simulink model "Robot_simulation2"  (R2025b)
settings: Solver=ode15s  StartTime=0.0  StopTime=Tf  FixedStep=dt  RelTol=1e-3
InitFcn:
  | run("init.m");
values from neighbouring files (symbols this model uses):
  dt = 0.1    [init.m]
  F_max = 1500    [init.m]
  F_min = 100    [init.m]
  g = in3(:,13)    [dinamica_3R_numerica.m]    (also in init.m = 9.81)
  k_d = diag([1000, 1000])    [init.m]
  k_p = diag([20000, 20000])    [init.m]
  L_max = 1.2    [init.m]
  mb = 66.5    [init.m]
  mu = 0.6    [init.m]
  N = 5    [init.m]
  q_init = cinematica_inversa_2R(0 , 0.6, robot_params)    [init.m]
  S_bar = 10*kron(eye(N), S)    [init.m]
  W_bar = kron(eye(N), W)    [init.m]
  x_ref = zeros(4, steps)    [init.m]
  x_ref_global = x_ref    [init.m]
undefined symbols (not defined in the file or in its folder): robot_params
libraries: simulink x2, slpidlib x1
settings Model: Creator=Acer  LastModifiedBy=Acer

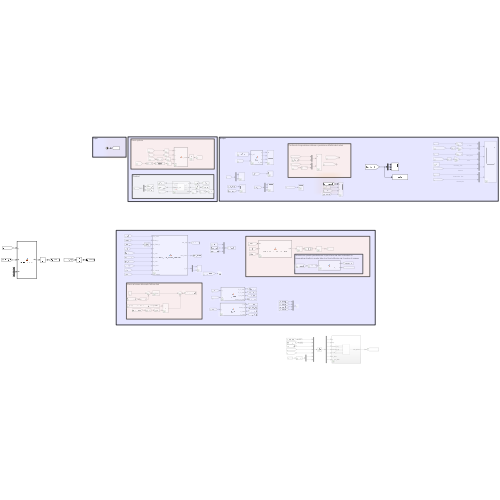
[thumbnail: Simulink's stored preview of the top-level diagram]
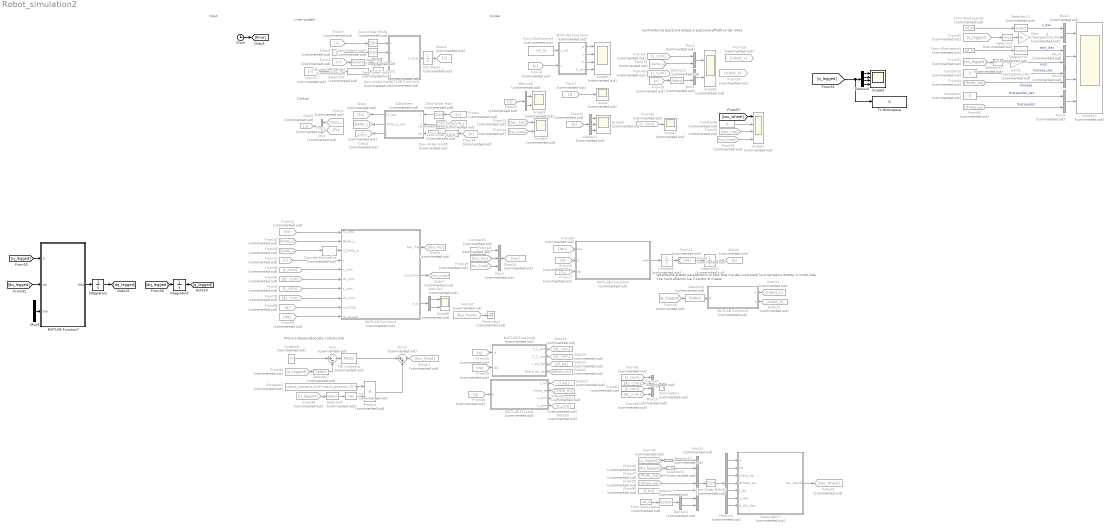
== system Robot_simulation2 ==
  note: Provo a tenere bloccato l'ultimo link
  note: Attenzione questo parallelismo lo puoi fare ma devi calcolarti la
      | cinematica diretta in modo tale che l'end effector sia il centro di massa
  note: Confronto tra posizione attesa e posizione effettiva del robot
  note: Control
  note: Liner system
  note: Input
  note: Scope
  Clock : Clock
  Constant{,3..6} (5 alike) : Constant  Commented=on  Value=0
  Constant2 : Constant  Commented=on  Value=robot_params.m3*robot_params.l3 *g
  Demux1 : Demux  Commented=on  Outputs=3
  Demux2 : Demux  Commented=on  Outputs=2
  Demux3 : Demux
  Demux4 : Demux  Commented=on  Outputs=2
  Demux5 : Demux  Commented=on  Outputs=2
  Demux6 : Demux  Commented=on  Outputs=7
  Discrete Derivative : simulink/Discrete/Discrete Derivative  Commented=on  gainval=1.0  ICPrevScaledInput=0.0  OutMin=[]  OutMax=[]  OutDataType=fixdt(1, 16)  OutScaling=2^-10  DoSatur=off
  Discrete Derivative1 : simulink/Discrete/Discrete Derivative  Commented=on  gainval=1.0  ICPrevScaledInput=0.0  OutMin=[]  OutMax=[]  OutDataType=fixdt(1, 16)  OutScaling=2^-10  DoSatur=off
  From : From  Commented=on  GotoTag=Fz
  From Workspace{1..3,5} (4 alike) : FromWorkspace  Commented=on  VariableName=ref_ts
  From{1,10,25,29} (4 alike) : From  Commented=on  GotoTag=Delta_s
  From11 : From  Commented=on  GotoTag=Fz
  From{2..4,6,12,26..28} (8 alike) : From  Commented=on  GotoTag=x
  From13 : From  Commented=on  GotoTag=tau_hip
  From14 : From  Commented=on  GotoTag=tau_knee
  From{15,17,39,69} (4 alike) : From  Commented=on  GotoTag=dq
  From{16,21..22,48,68} (5 alike) : From  Commented=on  GotoTag=q
  From18 : From  Commented=on  GotoTag=tau_hip
  From19 : From  Commented=on  GotoTag=tau_knee
  From20 : From  Commented=on  GotoTag=tau
  From23 : From  Commented=on  GotoTag=robot_x
  From24 : From  Commented=on  GotoTag=robot_h
  From{35..36,38,45,50} (5 alike) : From  Commented=on  GotoTag=q_legged
  From37 : From  Commented=on  GotoTag=tau_head
  From42 : From  Commented=on  GotoTag=s_com
  From{43,53,58,65} (4 alike) : From  Commented=on  GotoTag=z_com
  From46 : From  Commented=on  GotoTag=dq_legged
  From47 : From  Commented=on  GotoTag=theta_eq
  From49 : From  Commented=on  GotoTag=l_eq
  From5 : From  Commented=on  GotoTag=time
  From51 : From  Commented=on  GotoTag=dq_legged
  From54 : From  Commented=on  GotoTag=tau_hip
  From55 : From  Commented=on  GotoTag=tau_knee
  From56 : From  Commented=on  GotoTag=dtheta_eq
  From59 : From  Commented=on  GotoTag=ds_com
  From60 : From  Commented=on  GotoTag=dz_com
  From61 : From  Commented=on  GotoTag=s_com
  From62 : From  Commented=on  GotoTag=ds_com
  From63 : From  Commented=on  GotoTag=dtheta_eq
  From64 : From  Commented=on  GotoTag=theta_eq
  From66 : From  Commented=on  GotoTag=dz_com
  From67 : From  Commented=on  GotoTag=u
  From7 : From  Commented=on  GotoTag=J
  From8 : From  Commented=on  GotoTag=u
  From9 : From  Commented=on  GotoTag=s_com
  Gain : Gain  Commented=on  Gain=robot_params.Rw
  Gain1 : Gain  Commented=on  Gain=robot_params.Rw
  Goto : Goto  Commented=on  GotoTag=Fz
  Goto1 : Goto  Commented=on  GotoTag=Delta_s
  Goto10 : Goto  Commented=on  GotoTag=tau
  Goto11 : Goto  Commented=on  GotoTag=robot_x
  Goto12 : Goto  Commented=on  GotoTag=robot_h
  Goto13 : Goto  Commented=on  GotoTag=tau_head
  Goto16 : Goto  Commented=on  GotoTag=ds_com
  Goto17 : Goto  Commented=on  GotoTag=l_eq
  Goto18 : Goto  Commented=on  GotoTag=theta_eq
  Goto19 : Goto  Commented=on  GotoTag=s_com
  Goto2 : Goto  Commented=on  GotoTag=J
  Goto20 : Goto  Commented=on  GotoTag=z_com
  Goto21 : Goto  Commented=on  GotoTag=dl_eq
  Goto22 : Goto  Commented=on  GotoTag=tau_wheel
  Goto23 : Goto  Commented=on  GotoTag=dtheta_eq
  Goto24 : Goto  Commented=on  GotoTag=dz_com
  Goto4 : Goto  Commented=on  GotoTag=x
  Goto5 : Goto  Commented=on  GotoTag=u
  Goto6 : Goto  Commented=on  GotoTag=tau_hip
  Goto7 : Goto  Commented=on  GotoTag=tau_knee
  Goto8 : Goto  Commented=on  GotoTag=dq
  Goto9 : Goto  Commented=on  GotoTag=q
  Integrator : Integrator  Commented=on  InitialCondition=zeros(3,1)
  Integrator1 : Integrator  Commented=on  InitialCondition=[q_init;0]
  Integrator2 : Integrator  InitialCondition=zeros(4,1)
  Integrator3 : Integrator  InitialCondition=[0;q_init;0]
  MATLAB Function : MATLAB Function  Commented=on  TreatAsAtomicUnit=on
  MATLAB Function1 : MATLAB Function  Commented=on  TreatAsAtomicUnit=on
  MATLAB Function2 : MATLAB Function  Commented=on  TreatAsAtomicUnit=on
  MATLAB Function3 : MATLAB Function  Commented=on  TreatAsAtomicUnit=on
  MATLAB Function4 : MATLAB Function  Commented=on  TreatAsAtomicUnit=on
  MATLAB Function5 : MATLAB Function  Commented=on  TreatAsAtomicUnit=on
  MATLAB Function7 : MATLAB Function  TreatAsAtomicUnit=on
  MATLAB Function8 : MATLAB Function  Commented=on  TreatAsAtomicUnit=on
  Mux{,2..5,8..9} (7 alike) : Mux  Commented=on  Inputs=2
  Mux1 : Mux  Commented=on  Inputs=3
  Mux10 : Mux  Commented=on
  Mux11 : Mux  Commented=on  Inputs=[1 1 1 1 1 1 1]
  Mux6 : Mux  Inputs=[1 1 2]
  PID Controller : slpidlib/PID Controller  Commented=on  Controller=PID  Form=Parallel  TimeDomain=Continuous-time  UseExternalTs=off  SampleTime=-1  IntegratorMethod=Forward Euler  FilterMethod=Forward Euler  ControllerParametersSource=internal  P=10000  I=10  UseKiTs=off  D=10  UseExternalDerivativeSource=off  N=100  UseFilter=on  TunerSelectOption=Frequency Response Based  InitialConditionSource=internal  InitialConditionForIntegrator=0  InitialConditionForFilter=0  DifferentiatorICPrevScaledInput=0  ExternalReset=none  TrackingMode=off  Kt=1  LimitOutput=off  SatLimitsSource=internal  UpperSaturationLimit=inf  LowerSaturationLimit=-inf  LinearizeAsGain=on  AntiWindupMode=none  Kb=1  LimitIntegrator=off  UpperIntegratorSaturationLimit=inf  LowerIntegratorSaturationLimit=-inf  POutMin=[]  POutMax=[]  IOutMin=[]  IOutMax=[]  DOutMin=[]  DOutMax=[]  NOutMin=[]  NOutMax=[]  SumOutMin=[]  SumOutMax=[]  SaturationOutMin=[]  SaturationOutMax=[]  PParamMin=[]  PParamMax=[]  IParamMin=[]  IParamMax=[]  DParamMin=[]  DParamMax=[]  NParamMin=[]  NParamMax=[]  KbParamMin=[]  KbParamMax=[]  KtParamMin=[]  KtParamMax=[]  KbOutMin=[]  KbOutMax=[]  KtOutMin=[]  KtOutMax=[]  IntegratorOutMin=[]  IntegratorOutMax=[]  FilterOutMin=[]  FilterOutMax=[]  SumI1OutMin=[]  SumI1OutMax=[]  SumI2OutMin=[]  SumI2OutMax=[]  SumI3OutMin=[]  SumI3OutMax=[]  SumI4OutMin=[]  SumI4OutMax=[]  SumDOutMin=[]  SumDOutMax=[]  DifferentiatorOutMin=[]  DifferentiatorOutMax=[]  FilterDiffOutCoefMin=[]  FilterDiffOutCoefMax=[]  ReciprocalOutMin=[]  ReciprocalOutMax=[]  SumDenOutMin=[]  SumDenOutMax=[]  SumNumOutMin=[]  SumNumOutMax=[]  DivideOutMin=[]  DivideOutMax=[]  UdiffTsProdOutMin=[]  UdiffTsProdOutMax=[]  NTsProdOutMin=[]  NTsProdOutMax=[]  UintegralTsProdOutMin=[]  UintegralTsProdOutMax=[]  UngainTsProdOutMin=[]  UngainTsProdOutMax=[]  ClampingZeroOutDataTypeStr=Inherit: Inherit via back propagation  ClampingZeroOutMin=[]  ClampingZeroOutMax=[]  FilterDenConstantOutDataTypeStr=Inherit: Inherit via back propagation  FilterDenConstantOutMin=[]  FilterDenConstantOutMax=[]  PCopyOutDataTypeStr=Inherit: Inherit via back propagation  PCopyOutMin=[]  PCopyOutMax=[]  NCopyOutDataTypeStr=Inherit: Inherit via back propagation  NCopyOutMin=[]  NCopyOutMax=[]  IntegratorContinuousStateAttributes=''  IntegratorStateMustResolveToSignalObject=off  IntegratorRTWStateStorageClass=Auto  FilterContinuousStateAttributes=''  FilterStateMustResolveToSignalObject=off  FilterRTWStateStorageClass=Auto  ParallelPVariant=InternalParameters  IdealPVariant=Disabled  IVariant=InternalParameters  DVariant=InternalParameters  IntegratorVariant=Continuous  SatVariant=Disabled  AWVariant=Passthrough  PCopyVariant=Disabled  TRVariant=Disabled  FdbkBlocksVariant=Forward  IdealPFdbkVariant=Disabled  SatFdbkVariant=Disabled  DerivativeFilterVariant=ContFilter  NVariant=InternalParameters  NCopyVariant=Disabled  FilterICVariant=InternalICsFilter  IntegratorICVariant=InternalICs  ExternalResetVariant=Disabled  TRSumVariant=Passthrough  SumFdbkVariant=Disabled  SumVariant=Sum_PID  TsampFilterVariant=InternalTs  TsampNgainVariant=Passthrough  TsampIntegralVariant=Disabled_SignalSpec  ExternalSaturationOutDataTypeStr=Inherit: Same as second input  DerivativeSourceVariant=ErrorSignal  PreIntVariant=InternalPreInt
  Product : Product  Commented=on
  Scope : Scope  Commented=on
      settings: ActiveDisplayYMinimum=-1  ActiveDisplayYMaximum=1
  Scope1 : Scope  Commented=on  NumInputPorts=4
      settings: ActiveDisplayYMinimum=-1  ActiveDisplayYMaximum=1
  Scope10 : Scope  Commented=on  NumInputPorts=4
      settings: ActiveDisplayYMinimum=-17.232872762989807  ActiveDisplayYMaximum=4.2885654585543138  DataLoggingVariableName=ScopeData10
  Scope2 : Scope  Commented=on  NumInputPorts=4
      settings: ActiveDisplayYMinimum=-0.12515032259253614  ActiveDisplayYMaximum=1.1263529033328255  DataLoggingVariableName=ScopeData2
  Scope3 : Scope  NumInputPorts=4
      settings: ActiveDisplayYMinimum=-33.446881867150935  ActiveDisplayYMaximum=300.84907271752644  DataLoggingVariableName=ScopeData3
  Scope{4,6,8..9} (4 alike) : Scope  Commented=on  NumInputPorts=2
      Scope4 settings: ActiveDisplayYMinimum=-277.12659813654608  ActiveDisplayYMaximum=-227.4623965158911  DataLoggingVariableName=ScopeData4
      Scope6 settings: ActiveDisplayYMinimum=-1  ActiveDisplayYMaximum=1  DataLoggingVariableName=ScopeData6
      Scope8 settings: ActiveDisplayYMinimum=-0.17028433513177135  ActiveDisplayYMaximum=0.13336662971669377  DataLoggingVariableName=ScopeData8
      Scope9 settings: ActiveDisplayYMinimum=-0.0048922557383608324  ActiveDisplayYMaximum=0.0030434800856270639  DataLoggingVariableName=ScopeData9
  Scope5 : Scope  Commented=on  NumInputPorts=3
      settings: ActiveDisplayYMinimum=-1.5053334308874105  ActiveDisplayYMaximum=1.0672403229769873  DataLoggingVariableName=ScopeData5
  Scope7 : Scope  Commented=on
      settings: ActiveDisplayYMinimum=-1  ActiveDisplayYMaximum=1  DataLoggingVariableName=ScopeData7
  Selector : Selector  Commented=on  InputPortWidth=4  IndexOptions=Index vector (dialog)  Indices=[3]  OutputSizes=1
  Selector1 : Selector  Commented=on  InputPortWidth=4  IndexOptions=Index vector (dialog)  Indices=[1 2]  OutputSizes=1
  Selector{3,10..14} (6 alike) : Selector  Commented=on  InputPortWidth=4  IndexOptions=Index vector (dialog)  Indices=[1]  OutputSizes=1
  Selector2 : Selector  Commented=on  InputPortWidth=4  IndexOptions=Index vector (dialog)  Indices=[3]  OutputSizes=1
  Selector4 : Selector  Commented=on  InputPortWidth=4  IndexOptions=Index vector (dialog)  Indices=[2 3]  OutputSizes=1
  Selector5 : Selector  Commented=on  InputPortWidth=4  IndexOptions=Index vector (dialog)  Indices=[4]  OutputSizes=1
  Selector6 : Selector  Commented=on  InputPortWidth=4  IndexOptions=Index vector (dialog)  Indices=[3]  OutputSizes=1
  Selector7 : Selector  Commented=on  InputPortWidth=4  IndexOptions=Index vector (dialog)  Indices=[4]  OutputSizes=1
  Selector8 : Selector  Commented=on  InputPortWidth=4  IndexOptions=Index vector (dialog)  Indices=[4]  OutputSizes=1
  Sin : Trigonometry  Commented=on  Operator=cos
  Subsystem : Subsystem  Commented=on
  Subsystem1 : Subsystem  Commented=on
  Sum : Sum  Commented=on  Inputs=|+-
  Sum1 : Sum  Commented=on  Inputs=|++
  Terminator : Terminator  Commented=on
  Terminator1 : Terminator  Commented=on
  To Workspace : ToWorkspace  VariableName=q  SaveFormat=Timeseries  SampleTime=-1
  Unit Delay : UnitDelay  Commented=on  InitialCondition=x_ref(:,1)  SampleTime=dt  HasFrameUpgradeWarning=on
  Zero-Order Hold{,1..6} (7 alike) : ZeroOrderHold  Commented=on  SampleTime=dt
  Zero-Order Hold12 : ZeroOrderHold  Commented=on  SampleTime=dt*100
  wires:
  MATLAB Function1/1(x_next) -> Unit Delay/1
  Subsystem/1(Fz_opt) -> Goto/1
  Subsystem/2(Delta_s_opt) -> Goto1/1
  Subsystem/3(J) -> Goto2/1
  Clock/1 -> [time]
  From1/1 -> Mux/1
  From/1 -> Mux/2
  From2/1 -> Selector/1
  From5/1 -> Zero-Order Hold4/1
  From Workspace3/1 -> MATLAB Function2/1(x_ref)
  MATLAB Function2/2(v) -> Scope2/2
  MATLAB Function2/1(p) -> Scope2/1
  MATLAB Function2/3(h) -> Scope2/3
  MATLAB Function2/4(h_dot) -> Scope2/4
  From6/1 -> MATLAB Function2/2(x)
  From7/1 -> Scope/1
  Mux/1 -> Goto5/1
  From12/1 -> MATLAB Function3/4(x)
  From11/1 -> MATLAB Function3/1(Fz_cmd)
  MATLAB Function3/1(tau_hip) -> Goto6/1
  MATLAB Function3/2(tau_knee) -> Goto7/1
  From14/1 -> Scope4/2
  From13/1 -> Scope4/1
  MATLAB Function4/1(qdd) -> Integrator/1
  Integrator/1 -> Goto8/1
  From15/1 -> Integrator1/1
  Integrator1/1 -> Goto9/1
  From16/1 -> MATLAB Function4/2(q)
  From17/1 -> MATLAB Function4/3(dq)
  Constant5/1 -> Mux1/1
  From18/1 -> Mux1/2
  Mux1/1 -> Goto10/1
  From20/1 -> MATLAB Function4/1(tau)
  From21/1 -> Demux1/1
  Demux1/1 -> Scope5/1
  Demux1/2 -> Scope5/2
  MATLAB Function5/1(x) -> Goto11/1
  MATLAB Function5/2(z) -> Goto12/1
  From42/1 -> Mux2/1
  From25/1 -> Mux2/2
  From43/1 -> Mux3/1
  Selector2/1 -> Mux3/2
  Mux2/1 -> Scope8/1
  Mux3/1 -> Scope8/2
  From69/1 -> MATLAB Function3/10(dq_actual)
  From68/1 -> MATLAB Function3/9(q_actual)
  From26/1 -> Selector2/1
  Zero-Order Hold/1 -> Subsystem/1(x)
  From4/1 -> Zero-Order Hold/1
  From10/1 -> MATLAB Function3/2(Delta_s)
  From29/1 -> Discrete Derivative/1
  Discrete Derivative/1 -> MATLAB Function3/3(d_Delta_s)
  Zero-Order Hold1/1 -> MATLAB Function1/1(x)
  From3/1 -> Zero-Order Hold1/1
  Zero-Order Hold2/1 -> MATLAB Function1/2(u)
  From8/1 -> Zero-Order Hold2/1
  Selector/1 -> Zero-Order Hold3/1
  Zero-Order Hold3/1 -> MATLAB Function1/3(h)
  Zero-Order Hold4/1 -> Subsystem/2(t)
  MATLAB Function7/1(ddq) -> Integrator2/1
  [dq_legged] -> Integrator3/1
  Integrator2/1 -> [dq_legged]
  Demux3/4 -> Scope3/4
  Integrator3/1 -> [q_legged]
  [q_legged] -> MATLAB Function7/1(q)
  Demux3/3 -> Scope3/3
  Demux3/2 -> Scope3/2
  Demux3/1 -> Scope3/1
  Mux6/1 -> MATLAB Function7/3(tau)
  [dq_legged] -> MATLAB Function7/2(dq)
  From35/1 -> Selector4/1
  Selector4/1 -> MATLAB Function5/1(q)
  From36/1 -> Selector7/1
  Constant/1 -> Sum/1
  Selector7/1 -> Sum/2
  Sum/1 -> PID Controller/1
  PID Controller/1 -> Sum1/1
  Sum1/1 -> Goto13/1
  Constant2/1 -> Product/1
  Product/1 -> Sum1/2
  Sin/1 -> Product/2
  From38/1 -> Selector8/1
  Selector8/1 -> Sin/1
  From48/1 -> MATLAB Function/1(q)
  MATLAB Function/1(l_eq) -> Goto17/1
  MATLAB Function/2(theta_eq) -> Goto18/1
  MATLAB Function/3(s_com) -> Goto19/1
  MATLAB Function/4(z_com) -> Goto20/1
  Zero-Order Hold5/1 -> Subsystem/3(zb)
  Selector6/1 -> Zero-Order Hold5/1
  MATLAB Function3/3(p_d) -> Demux2/1
  Demux2/1 -> Scope6/1
  Demux2/2 -> Scope6/2
  [q_legged] -> To Workspace/1, Demux3/1
  From53/1 -> Scope7/1
  From22/1 -> MATLAB Function8/1(q)
  MATLAB Function8/1(S_C_dot) -> Goto16/1
  MATLAB Function8/3(l_eq_dot) -> Goto21/1
  MATLAB Function8/4(theta_eq_dot) -> Goto23/1
  MATLAB Function8/2(Z_C_dot) -> Goto24/1
  From39/1 -> MATLAB Function8/2(dq)
  From Workspace1/1 -> Selector1/1
  Selector1/1 -> Demux4/1
  From50/1 -> Selector3/1
  From51/1 -> Selector10/1
  From Workspace2/1 -> Selector11/1
  Selector3/1 -> Gain/1
  Selector10/1 -> Gain1/1
  Selector11/1 -> Mux4/1  "s_des"
  Gain/1 -> Mux4/2  "s"
  Selector12/1 -> Mux5/1  "sdot_des"
  Gain1/1 -> Mux5/2  "sdot"
  Mux4/1 -> Scope10/1
  Mux5/1 -> Scope10/2
  From58/1 -> MATLAB Function3/5(z_com)
  From9/1 -> MATLAB Function3/7(s_com)
  From60/1 -> MATLAB Function3/6(dz_com)
  From59/1 -> MATLAB Function3/8(ds_com)
  Mux9/1 -> Scope10/4
  Mux8/1 -> Scope10/3
  From63/1 -> Mux9/2  "thetaeqdot"
  Constant4/1 -> Mux9/1  "thetaeqdot_des"
  From64/1 -> Mux8/2  "thetaeq"
  Constant3/1 -> Mux8/1  "thetaeq_des"
  From61/1 -> Mux10/1
  From62/1 -> Mux10/2
  From65/1 -> Mux10/3
  From66/1 -> Mux10/4
  Mux10/1 -> Terminator1/1
  Demux5/2 -> Scope9/2
  Demux5/1 -> Scope9/1
  From67/1 -> Demux5/1
  Unit Delay/1 -> Goto4/1
  From45/1 -> Selector13/1
  From46/1 -> Selector14/1
  Subsystem1/1(tau_wheel) -> Goto22/1
  Selector13/1 -> Mux11/1
  Selector14/1 -> Mux11/2
  From47/1 -> Mux11/3
  From56/1 -> Mux11/4
  From49/1 -> Mux11/5
  Demux4/1 -> Mux11/6
  Demux4/2 -> Mux11/7
  Mux11/1 -> Zero-Order Hold12/1
  Zero-Order Hold12/1 -> Demux6/1
  Demux6/1 -> Subsystem1/1(q)
  Demux6/2 -> Subsystem1/2(dq)
  Demux6/3 -> Subsystem1/3(theta_eq)
  Demux6/4 -> Subsystem1/4(dtheta_eq)
  Demux6/5 -> Subsystem1/5(l_eq)
  Demux6/6 -> Subsystem1/6(s_des)
  Demux6/7 -> Subsystem1/7(s_dot_des)
  From Workspace5/1 -> Selector12/1
  From37/1 -> Terminator/1
  From19/1 -> Mux1/3
  [tau_wheel] -> Scope1/1
  Constant6/1 -> Scope1/2
  From54/1 -> Scope1/3
  From55/1 -> Scope1/4
  Demux1/3 -> Scope5/3
  From28/1 -> Selector6/1
  Discrete Derivative1/1 -> Zero-Order Hold6/1
  From27/1 -> Selector5/1
  Selector5/1 -> Discrete Derivative1/1
  Zero-Order Hold6/1 -> MATLAB Function1/4(ddz)

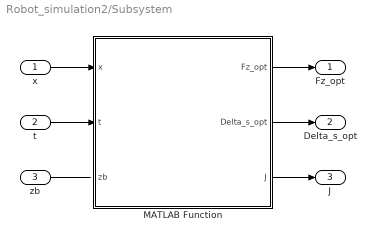
== system Robot_simulation2/Subsystem ==
  x : Inport
  t : Inport  Port=2
  zb : Inport  Port=3
  MATLAB Function : MATLAB Function  TreatAsAtomicUnit=on
  Fz_opt : Outport
  Delta_s_opt : Outport  Port=2
  J : Outport  Port=3
  wires:
  x/1 -> MATLAB Function/1(x)
  MATLAB Function/1(Fz_opt) -> Fz_opt/1
  MATLAB Function/2(Delta_s_opt) -> Delta_s_opt/1
  MATLAB Function/3(J) -> J/1
  t/1 -> MATLAB Function/2(t)
  zb/1 -> ?

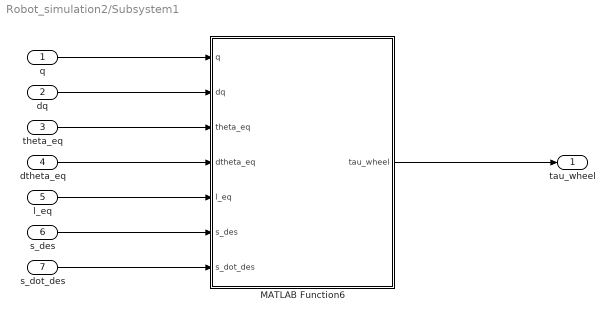
== system Robot_simulation2/Subsystem1 ==
  q : Inport
  dq : Inport  Port=2
  theta_eq : Inport  Port=3
  dtheta_eq : Inport  Port=4
  l_eq : Inport  Port=5
  s_des : Inport  Port=6
  s_dot_des : Inport  Port=7
  MATLAB Function6 : MATLAB Function  TreatAsAtomicUnit=on
  tau_wheel : Outport
  wires:
  dtheta_eq/1 -> MATLAB Function6/4(dtheta_eq)
  l_eq/1 -> MATLAB Function6/5(l_eq)
  s_dot_des/1 -> MATLAB Function6/7(s_dot_des)
  q/1 -> MATLAB Function6/1(q)
  theta_eq/1 -> MATLAB Function6/3(theta_eq)
  dq/1 -> MATLAB Function6/2(dq)
  s_des/1 -> MATLAB Function6/6(s_des)
  MATLAB Function6/1(tau_wheel) -> tau_wheel/1

== matlab function Robot_simulation2/MATLAB Function5 ==
  data: q input; x output; z output; robot_params parameter
function [x,z] = cinematica_diretta(q,robot_params)


[x,z] = cinematica_diretta_2R(q, robot_params);

== matlab function Robot_simulation2/MATLAB Function ==
  data: q input size=3; l_eq output; theta_eq output; s_com output; z_com output; robot_params parameter
function [l_eq,theta_eq, s_com, z_com] = CoM(q,robot_params)

[l_eq,theta_eq, s_com, z_com] = calcola_CoM_equivalente(q, robot_params);

end

== matlab function Robot_simulation2/MATLAB Function7 ==
  data: q input; ddq output size=4; dq input; tau input
function ddq =  whole_robot_2D(q, dq, tau)
    % tau è il vettore delle coppie/forze generalizzate in ingresso (4x1)
    
    % 1. Calcola le matrici dinamiche valutate nello stato attuale
    [M, C, G] = Dinamica_Robot(q, dq);
    
    % 2. Risolvi l'equazione del moto: M*ddq + C*dq + G = tau
    % In MATLAB/Simulink si usa l'operatore mldivide (\) per invertire M in modo robusto
    ddq = M \ (tau - C*dq - G);
end

== matlab function Robot_simulation2/Subsystem1/MATLAB Function6 ==
  data: q input; tau_wheel output; dq input; theta_eq input; dtheta_eq input; l_eq input; s_des input; s_dot_des input; robot_params parameter
function tau_wheel  = TV_LQR_Online(q, dq, theta_eq, dtheta_eq, l_eq, s_des, s_dot_des, robot_params)
    % Comando magico per poter usare lqr() dentro Simulink senza errori di compilazione
    coder.extrinsic('lqr');

    
    % --- PROTEZIONE DA DIVISIONE PER ZERO ---
    %l_eq = max(l_eq, 0.4); 
    
    % --- 1. Estrazione Parametri Fisici dalla Struct ---
    m_w = robot_params.mw;      
    I_w = robot_params.Iw;      
    r   = robot_params.Rw;           
    m_b = robot_params.mb; 
    g   = 9.81;
    
    % --- 2. Costruzione Stato (X) e Riferimento (X_des) ---
    % Adesso lo stato è a 4 variabili: [s; theta_eq; s_dot; theta_dot]
    s = q * r;
    s_dot = dq * r;
    X = [s; theta_eq; s_dot; dtheta_eq];
    
    X_des = [s_des; 0; s_dot_des; 0];
    
    % --- 3. Ricalcolo Dinamico Matrici A (4x4) e B (4x1) ---
    I_y = (1/3) * m_b * l_eq^2;
    
    % Denominatore adattato per UNA SOLA ruota (tolti i '2*')
    den = I_w*(I_y + m_b*l_eq^2) + (l_eq^2*m_b*m_w + I_y*(m_b + m_w)*r^2);
    
    % Coefficienti adattati per UNA SOLA ruota
    a_1 = - (g * l_eq^2 * m_b^2 * r^2) / den;
    a_2 = (g * l_eq * m_b * (I_w + (m_b + m_w)*r^2)) / den;
    b_1 = (r * (I_y + l_eq*m_b*(l_eq + r))) / den;
    b_2 = - (I_w + r*(l_eq*m_b + (m_b + m_w)*r)) / den;
    
    A = zeros(4,4);
    A(1,3) = 1; 
    A(2,4) = 1; 
    A(3,2) = a_1;
    A(4,2) = a_2;
    
    B = zeros(4,1);
    B(3,1) = b_1; 
    B(4,1) = b_2; 
    
% --- 4. Calcolo LQR Online ---
    % Rimettiamo un peso > 0 sulla posizione (es. 10) per garantire la rilevabilità
    %Q = diag([1000, 1, 0.1, .1]); 
    Q = diag([200, .01, 1, .1]); 
    R = 100;
    
    K = zeros(1, 4); 
    K = lqr(A, B, Q, R); % Ora non darà più errore!
    
    % --- 5. Azione di Controllo (Inseguimento Traiettoria Reale) ---
    % L'errore è (Stato_attuale - Riferimento)
    X_error = [ (s - s_des); 
                (theta_eq - 0); 
                (s_dot - s_dot_des); 
                (dtheta_eq - 0) ];
    
    tau_wheel =K * X_error;
end

== matlab function Robot_simulation2/MATLAB Function8 ==
  data: q input; dq input; S_C_dot output; Z_C_dot output; l_eq_dot output; theta_eq_dot output; robot_params parameter
function [S_C_dot, Z_C_dot, l_eq_dot, theta_eq_dot] = J_CoM(q,dq,robot_params)
    %#codegen
    % CALCOLA_VELOCITA_COM_SIMULINK Calcola le velocità del CoM e del pendolo 
    % equivalente (WIP) per l'utilizzo in Simulink.
    
    % --- 1. Estrazione Variabili di Stato ---
    q1 = q(1);
    q2 = q(1);
    q3 = q(2);
    
    % --- 2. Estrazione Parametri Robot ---
    l1 = robot_params.l1;
    l2 = robot_params.l2;
    l3 = robot_params.l3;
    
    m1 = robot_params.m1;
    m2 = robot_params.m2;
    m3 = robot_params.m3;
    m_upper = m1 + m2 + m3;
    
    % --- 3. Costanti Raggruppate per l'Analitica ---
    K1 = (m1 * (l1/2) + m2 * l1 + m3 * l1) / m_upper;
    K2 = (m2 * (l2/2) + m3 * l2) / m_upper;
    K3 = (m3 * (l3/2)) / m_upper;
    
    % --- 4. Ricalcolo Posizione CoM ---
    S_C = K1*cos(q1) + K2*cos(q1+q2) + K3*sin(q3);
    Z_C = K1*sin(q1) + K2*sin(q1+q2) + K3*cos(q3);
    
    % --- 5. Calcolo Jacobiano (J_CoM) ---
    % Preallocazione statica della matrice 2x4 per compatibilità C/C++
    J_CoM = zeros(2, 3);
    
    % Derivate parziali di S_C (Prima Riga)
    J_CoM(1, 1) = -K1*sin(q1) - K2*sin(q1+q2);
    J_CoM(1, 2) = -K2*sin(q1+q2);
    J_CoM(1, 3) =  K3*cos(q3);
    
    % Derivate parziali di Z_C (Seconda Riga)
    J_CoM(2, 1) =  K1*cos(q1) + K2*cos(q1+q2);
    J_CoM(2, 2) =  K2*cos(q1+q2);
    J_CoM(2, 3) = -K3*sin(q3);
    
    % --- 6. Calcolo Velocità Cartesiane ---
    % V_C = [S_C_dot; Z_C_dot]
    V_C = J_CoM * dq;
    S_C_dot = V_C(1);
    Z_C_dot = V_C(2);
    
    % --- 7. Derivate del Pendolo Equivalente e Gestione Singolarità ---
    l_eq_sq = S_C^2 + Z_C^2;
    l_eq = sqrt(l_eq_sq);
    

        l_eq_dot = (S_C * S_C_dot + Z_C * Z_C_dot) / l_eq;
        theta_eq_dot = (S_C_dot * Z_C - S_C * Z_C_dot) / l_eq_sq;
   end

== matlab function Robot_simulation2/MATLAB Function1 ==
  data: x input size=4; x_next output size=4; u input size=2; h input size=1; ddz input; g parameter; mb parameter; dt parameter
function x_next = fcn(x,u,h,ddz, g, mb,dt)

dc = [0; 0; 0; -g];     % Disturbo di gravità
dk = dc * dt;

Ac = [0 1 0 0; 0 0 0 0; 0 0 0 1; 0 0 0 0];
Bc = [0 0; (g+ddz)/h 0; 0 0; 0 1/mb];

    Ak = eye(4) + Ac * dt;
    Bk = Bc * dt;

   %dk disturbo di gravita
x_next = Ak*x + Bk*u + dk;

== matlab function Robot_simulation2/Subsystem/MATLAB Function ==
  data: x input; t input; g parameter; mb parameter; Fz_opt output; Delta_s_opt output; J output; dt parameter; mu parameter; W_bar parameter; S_bar parameter; F_max parameter; F_min parameter; N parameter; L_max parameter; x_ref_global parameter; zb input
function [Fz_opt, Delta_s_opt, J] = MPC(x,t,...              %INPUT
                                    g, mb, dt, mu, W_bar, S_bar, F_max, F_min, N, L_max, x_ref_global, zb) %PARAMETERS

    steps_totali = size(x_ref_global, 2);
    
    % Calcolo dell'indice attuale k basato sul tempo
    % Aggiungiamo 1 perché MATLAB usa indici che partono da 1 (t=0 -> k=1)
    k_curr = floor(t / dt) + 1; 
    
    % Inizializza il vettore per l'orizzonte N
    X_ref_window = zeros(4*N, 1);
    
    for i = 1:N
        % Calcola l'indice futuro. Il "min" serve come saturazione: 
        % se l'orizzonte guarda oltre la fine della simulazione, tiene l'ultimo target.
        idx = min(k_curr + i - 1, steps_totali); 
        
        % Inserisce i 4 stati futuri nello slot corretto
        X_ref_window((i-1)*4+1 : i*4) = x_ref_global(:, idx);
    end
    
    h_k = x(3);
    dc = [0; 0; 0; -g];     % Disturbo di gravità
    dk = dc * dt;
    
    % --- Ricalcolo Dinamica Locale basata su h_k ---
    Ac = [0 1 0 0; 0 0 0 0; 0 0 0 1; 0 0 0 0];
    Bc = [0 0; g/h_k 0; 0 0; 0 1/mb];
    Ak = eye(4) + Ac * dt;
    Bk = Bc * dt;
    
    % --- Aggiornamento Dinamico dei Vincoli ---
    max_kinematic_ds = sqrt(L_max^2 - zb^2);
    ds_min = max(-mu*h_k, -max_kinematic_ds);
    ds_max = min(mu*h_k, max_kinematic_ds);
    
    U_min = [ds_min; F_min];
    U_max = [ds_max; F_max];
    LB = repmat(U_min, N, 1);
    UB = repmat(U_max, N, 1);
    
    % --- Calcolo Matrici di Predizione per l'orizzonte N ---
    Phi = zeros(4*N, 2*N);
    Psi = zeros(4*N, 4);
    Term_dist = zeros(4*N, 1);
    
    for i = 1:N
        Psi((i-1)*4+1:i*4, :) = Ak^i;
        for j = 1:i
            Phi((i-1)*4+1:i*4, (j-1)*2+1:j*2) = (Ak^(i-j)) * Bk;
            Term_dist((i-1)*4+1:i*4) = Term_dist((i-1)*4+1:i*4) + (Ak^(i-j))*dk;
        end
    end
    
    H = 2 * (Phi' * S_bar * Phi + W_bar);
    f = 2 * Phi' * S_bar * (Psi * x + Term_dist - X_ref_window);

 % --- 5. RISOLUZIONE QP ---
    options = optimoptions('quadprog', 'Algorithm', 'active-set', 'Display', 'off');
    
    % Definisci l'ingresso di equilibrio (Delta_s = 0, F_z = massa * gravità)
    u_guess_step = [0; mb * g];
    
    % Replicato per tutto l'orizzonte N
    U0_guess = repmat(u_guess_step, N, 1);
    
    % Passa U0_guess come 9° argomento invece di []
    [U_seq, fval] = quadprog(H, f, [], [], [], [], LB, UB,U0_guess,options);
    

    
    % --- Calcolo del vero costo ---
    Errore_non_controllato = (Psi * x + Term_dist - X_ref_window);
    cost_costante = Errore_non_controllato' * S_bar * Errore_non_controllato;
    J = fval + cost_costante;
    
    % --- Assegnazione Output Corretta ---
    u_opt = U_seq(1:2);
    Delta_s_opt = u_opt(1); % u_1 controlla la dinamica x
    Fz_opt = u_opt(2);      % u_2 controlla la dinamica z

end

== matlab function Robot_simulation2/MATLAB Function2 ==
  data: x_ref input; p output; x input; v output; h output; h_dot output
function [p, v, h, h_dot] = fcn(x_ref,x)

p = [x_ref(1),x(1)];
v = [x_ref(2),x(2)];
h = [x_ref(3),x(3)];
h_dot = [x_ref(4),x(4)];

== matlab function Robot_simulation2/MATLAB Function3 ==
  data: Fz_cmd input; Delta_s input; d_Delta_s input; tau_hip output; x input; z_com input; dz_com input; s_com input; ds_com input; k_p parameter; k_d parameter; tau_knee output; robot_params parameter; q_actual input; dq_actual input; p_d output
function [tau_hip, tau_knee, p_d] = new_Task_space_controller(Fz_cmd, Delta_s, d_Delta_s, x, z_com, dz_com, s_com, ds_com, k_p, k_d, robot_params, q_actual, dq_actual)
    
    % 1. Lettura dello stato REALE del robot
    t1 = q_actual(1);
    t2 = q_actual(2);
    t3 = q_actual(3);
    
    % Estrazione lunghezze dei link
    l1 = robot_params.l1;
    l2 = robot_params.l2;
    l3 = robot_params.l3;
    
    % Somme degli angoli (configurazioni assolute)
    t12  = t1 + t2;
    t123 = t1 + t2 + t3;
    
    %% 2. Calcolo Jacobiano Lineare (2x3) per coordinate cartesiane [X; Y]
    % Riga 1: Velocità lineare X
    j11 = -l1*sin(t1) - l2*sin(t12) - l3*sin(t123);
    j12 = -l2*sin(t12) - l3*sin(t123);
    j13 = -l3*sin(t123);
    
    % Riga 2: Velocità lineare Y
    j21 = l1*cos(t1) + l2*cos(t12) + l3*cos(t123);
    j22 = l2*cos(t12) + l3*cos(t123);
    j23 = l3*cos(t123);
    
    % Matrice Jacobiana Lineare
    J_L = [j11, j12, j13;
           j21, j22, j23];
    
    %% 3. Estrazione dello Jacobiano Attivo per i giunti 2 e 3
    % Escludiamo la prima colonna perché il giunto 1 non ha attuatore
    J_active = J_L(:, 2:3); % Matrice 2x2
    
    %% 4. Calcolo Errori e Forze nel Task Space
    % Posizione e velocità effettive (2x1)
    p_f = [s_com; z_com];     
    v_f = [ds_com; dz_com]; 
    
    % Posizione e velocità desiderate (2x1)
    p_d = [Delta_s; x(3)];
    v_d = [d_Delta_s; x(4)]; 
    
    % Forza di feedback
    F_feedback = k_p * (p_d - p_f) + k_d * (v_d - v_f);
    
    % Forza di feedforward
    F_feedforward = [0; Fz_cmd]; 
    
    % Forza totale richiesta nel Task Space
    F_tot = F_feedback + F_feedforward;
    
    %% 5. Mapping delle Coppie sui soli giunti attivi
    % tau_active conterrà [tau_giunto2; tau_giunto3]
    tau_active = J_active' * F_tot;
    
    % Assegnazione output (il giunto 1 ha coppia ZERO, non modificabile)
    tau_hip  = tau_active(1); % Coppia del giunto 2
    tau_knee = tau_active(2); % Coppia del giunto 3
end

== matlab function Robot_simulation2/MATLAB Function4 ==
  data: tau input; q input; qdd output; dq input; robot_params parameter; g parameter
function qdd = dinamica_robot_3R_con_carico(tau, q, dq, robot_params, g)
    % Carico applicato sull'end-effector (kg)
    mL = 70; 
    
    % Estrazione variabili di stato (angoli, velocità)
    theta1  = q(1);  theta2  = q(2);  theta3  = q(3);
    dtheta1 = dq(1); dtheta2 = dq(2); dtheta3 = dq(3);
    
    % Estrazione parametri del robot 3R
    m1 = robot_params.m1;   m2 = robot_params.m2;   m3 = robot_params.m3;
    l1 = robot_params.l1;   l2 = robot_params.l2;   l3 = robot_params.l3;
    lc1 = robot_params.l1/2; lc2 = robot_params.l2/2; lc3 = robot_params.l3/2;
    I1 = robot_params.I1;   I2 = robot_params.I2;   I3 = robot_params.I3;
    
    % Abbreviazioni trigonometriche per leggibilità
    s2   = sin(theta2);          c2   = cos(theta2);
    s3   = sin(theta3);          c3   = cos(theta3);
    s23  = sin(theta2 + theta3); c23  = cos(theta2 + theta3);
    
    %% 1. Matrice di Inerzia B(q)
    % Contributi accoppiati e termini di massa/inerzia equivalenti
    mu3 = m3*lc3 + mL*l3;
    mu2 = m2*lc2 + (m3 + mL)*l2;
    mu1 = m1*lc1 + (m2 + m3 + mL)*l1;
    
    b11 = I1 + I2 + I3 + m1*lc1^2 + m2*(l1^2 + lc2^2) + m3*(l1^2 + l2^2 + lc3^2) + mL*(l1^2 + l2^2 + l3^2) ...
          + 2*l1*mu2*c2 + 2*l2*mu3*c3 + 2*l1*mu3*c23;
          
    b12 = I2 + I3 + m2*lc2^2 + m3*(l2^2 + lc3^2) + mL*(l2^2 + l3^2) ...
          + l1*mu2*c2 + 2*l2*mu3*c3 + l1*mu3*c23;
          
    b13 = I3 + m3*lc3^2 + mL*l3^2 + l2*mu3*c3 + l1*mu3*c23;
    
    b21 = b12;
    b22 = I2 + I3 + m2*lc2^2 + m3*(l2^2 + lc3^2) + mL*(l2^2 + l3^2) + 2*l2*mu3*c3;
    b23 = I3 + m3*lc3^2 + mL*l3^2 + l2*mu3*c3;
    
    b31 = b13;
    b32 = b23;
    b33 = I3 + m3*lc3^2 + mL*l3^2;
    
    B = [b11, b12, b13; 
         b21, b22, b23; 
         b31, b32, b33];
         
    %% 2. Matrice di Coriolis e forze centrifughe C(q, dq)
    % Coefficienti di Christoffel semplificati analiticamente
    h1 = l1*mu2*s2 + l1*mu3*s23;
    h2 = l2*mu3*s3;
    h3 = l1*mu3*s23;
    
    c11 = -h1*dtheta2 - h3*dtheta3;
    c12 = -h1*(dtheta1 + dtheta2) - h2*dtheta3 - h3*dtheta3;
    c13 = -(h2 + h3)*(dtheta1 + dtheta2 + dtheta3);
    
    c21 = h1*dtheta1 - h2*dtheta3;
    c22 = -h2*dtheta3;
    c23 = -h2*(dtheta1 + dtheta2 + dtheta3);
    
    c31 = (h2 + h3)*dtheta1 + h2*dtheta2;
    c32 = h2*(dtheta1 + dtheta2);
    c33 = 0;
    
    C = [c11, c12, c13;
         c21, c22, c23;
         c31, c32, c33];
         
    %% 3. Vettore di Gravità G(q)
    % Calcolato assumendo lo zero della gravità lungo l'asse orizzontale (coseno)
    % coerentemente con il tuo script originale 2R.
    g1 = mu1*g*cos(theta1) + mu2*g*cos(theta1 + theta2) + mu3*g*cos(theta1 + theta2 + theta3);
    g2 = mu2*g*cos(theta1 + theta2) + mu3*g*cos(theta1 + theta2 + theta3);
    g3 = mu3*g*cos(theta1 + theta2 + theta3);
    
    G = [g1; g2; g3];
    
    %% Risoluzione dell'accelerazione
    qdd = B \ (tau - C*dq - G);
end
